simulink model "danxiangjiangya_org"  (Simulink 10.0)
settings: Solver=ode15s  StartTime=0.0  StopTime=0.05  RelTol=1e-3  EnableMultiTasking=on
libraries: powerlib x10, powerlib_extras x1
settings Model: Creator=Administrator  LastModifiedBy=bhisma
settings DataIOCC: LimitDataPoints=on  SignalLoggingSaveFormat=ModelDataLogs
settings OptimizationCC: BooleanDataType=off  InitFltsAndDblsToZero=on
settings DebuggingCC: SaveWithParameterizedLinksMsg=none  SignalResolutionControl=TryResolveAllWithWarning  MultiTaskDSMMsg=warning  MultiTaskCondExecSysMsg=none  FcnCallInpInsideContextMsg=warning  AllowSymbolicDim=off
settings HardwareCC: TargetUnknown=on
settings GRTTargetCC: TargetFcnLib=ansi_tfl_tmw.mat
settings ConfigComp: CovExternalEMLEnable=off
settings SimscapeCC: SimscapeNormalizeSystem=off

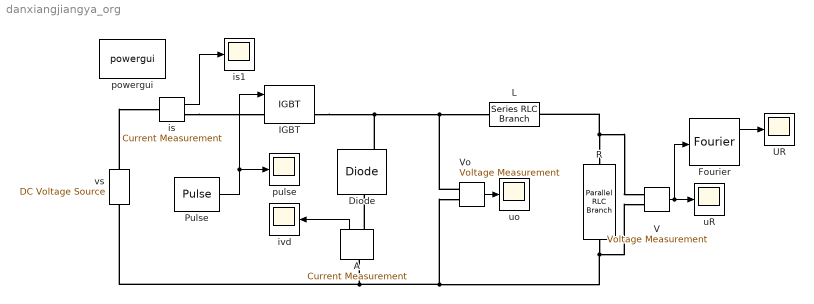
== system danxiangjiangya_org ==
  A : powerlib/Measurements/Current Measurement  PhasorSimulation=off  OutputType=Magnitude  PSBequivalent=0
      settings: SourceProductName=Simscape Electrical
  Diode : powerlib/Power Electronics/Diode  Ron=0.01  Lon=0  Vf=0.8  IC=0  UseSnubber=off  Rs=10  Cs=0.01e-6  Measurements=on
      settings: SourceProductName=Simscape Electrical
  Fourier : powerlib_extras/Measurements/Fourier  f1=500  n=0
      settings: SourceProductName=Simscape Electrical  SourceProductBaseCode=PS
  IGBT : powerlib/Power Electronics/IGBT  Ron=0.01  Lon=1e-6  Vf=1  Tf=1e-6  Tt=2e-6  IC=0  Rs=0  Cs=0.01e-6  Measurements=on
      settings: SourceProductName=Simscape Electrical
  "L " : powerlib/Elements/Series RLC Branch  LConnTagsString=__new0  RConnTagsString=__new0  BranchType=L  Resistance=[]  Inductance=1e-3  SetiL0=off  InitialCurrent=0  Capacitance=[]  Setx0=off  InitialVoltage=0  Measurements=None
      settings: SourceProductName=Simscape Electrical
  "Pulse " : DiscretePulseGenerator  PulseType=Time based  Period=0.002  PulseWidth=50
  R : powerlib/Elements/Parallel RLC Branch  LConnTagsString=a  RConnTagsString=__new0  BranchType=R  Resistance=1  Inductance=[]  SetiL0=off  InitialCurrent=0  Capacitance=[]  Setx0=off  InitialVoltage=0  Measurements=None
      settings: SourceProductName=Simscape Electrical
  UR : Scope
  V : powerlib/Measurements/Voltage Measurement  PhasorSimulation=off  OutputType=Magnitude  PSBequivalent=0
      settings: SourceProductName=Simscape Electrical
  Vo : powerlib/Measurements/Voltage Measurement  PhasorSimulation=off  OutputType=Magnitude  PSBequivalent=0
      settings: SourceProductName=Simscape Electrical
  is : powerlib/Measurements/Current Measurement  PhasorSimulation=off  OutputType=Magnitude  PSBequivalent=0
      settings: SourceProductName=Simscape Electrical
  is1 : Scope
  ivd : Scope
  powergui : powerlib/powergui  Priority=1  SimulationMode=Continuous  SampleTime=50e-6  frequency=60  Iterations=50  frequencyindice=0  Pbase=100e6  ErrMax=1e-4  UnitsV=kV  UnitsW=MW  buscounter=0  FunctionMessages=off  echomessages=off  EnableUseOfTLC=off  CurrentSourceSwitches=off  DisableSnubberDevices=off  DisableRonSwitches=off  DisableVfSwitches=off  DisplayEquations=off  AutomaticDiscreteSolvers=off  SolverType=Tustin/Backward Euler (TBE)  Interpol=off  ExternalGateDelay=off  methode=off  Ts=10  x0status=blocks  SPID=off  SwTol=0  HookPort=off  NonlinearTolerance=1e-4  nMaxIteration=100  ContinueOnMaxIteration=off  RestoreLinks=warning  ResistiveCurrentMeasurement=off  Frange=[0:2:500]  Ylog=off  Xlog=on  ShowGrid=off  save=off  variable=ZData  structure=0  ZoomFFT=off  StartTime=0.0  cycles=1  DisplayStyle=1  fundamental=60  FreqAxis=off  MaxFrequency=1000  frequencyindicesteady=1  RmsSteady=1  display=off
      settings: SourceProductName=Simscape Electrical
  pulse : Scope
  uR : Scope
  uo : Scope
  vs : powerlib/Electrical Sources/DC Voltage Source  Amplitude=200  Measurements=None
      settings: SourceProductName=Simscape Electrical
  wires:
  V/1 -> uR/1, Fourier/1
  A/1 -> ivd/1
  is/1 -> is1/1
  Vo/1 -> uo/1
  "Pulse "/1 -> IGBT/1, pulse/1
  Fourier/1 -> UR/1
  connections:
  vs/LConn1 -- A/LConn1 -- Vo/LConn2 -- R/RConn1 -- V/LConn2
  A/RConn1 -- Diode/LConn1
  vs/RConn1 -- is/LConn1
  is/RConn1 -- IGBT/LConn1
  IGBT/RConn1 -- Vo/LConn1 -- "L "/LConn1 -- Diode/RConn1
  "L "/RConn1 -- R/LConn1 -- V/LConn1
